simulink model "Lane_Keep_Assist"  (R2025a)
settings: Solver=VariableStepAuto  StartTime=0.0  StopTime=10.0  RelTol=1e-3
libraries: slpidlib x1
settings Model: Creator=Rudransh  LastModifiedBy=Rudransh

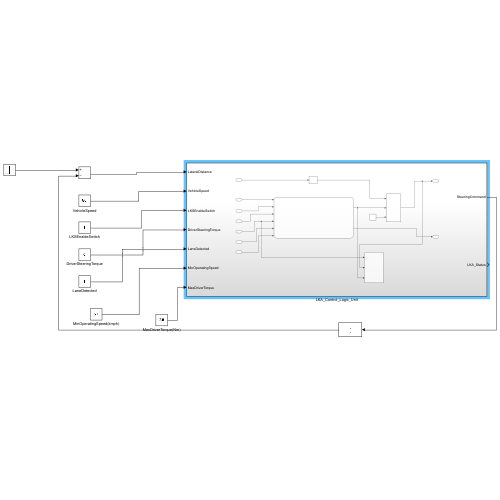
[thumbnail: Simulink's stored preview of the top-level diagram]
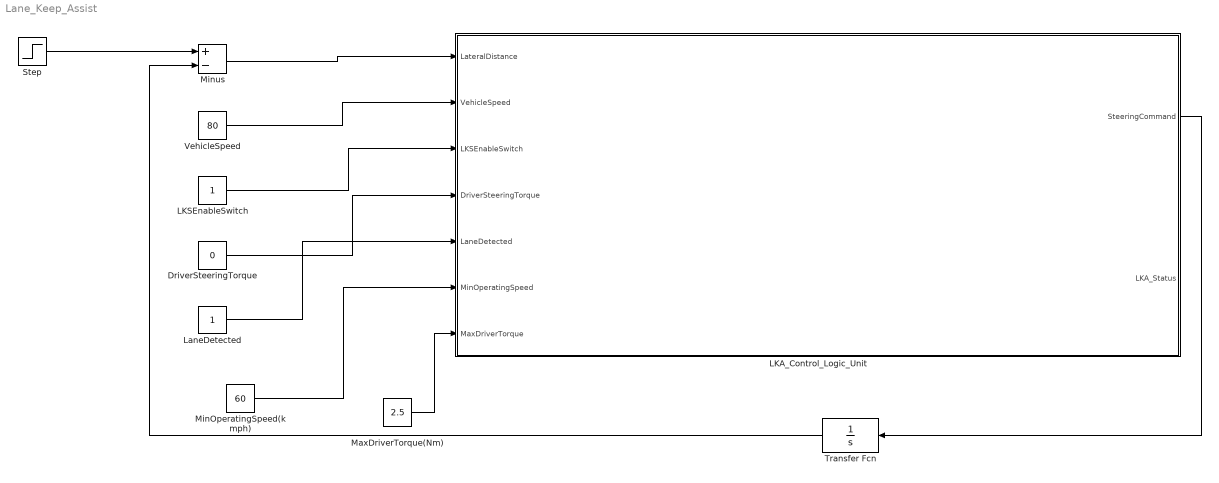
== system Lane_Keep_Assist ==
  DriverSteeringTorque : Constant  Value=0
  LKA_Control_Logic_Unit : Subsystem
  LKSEnableSwitch : Constant
  LaneDetected : Constant
  MaxDriverTorque(Nm) : Constant  Value=2.5
  MinOperatingSpeed(kmph) : Constant  Value=60
  Minus : Sum  Inputs=+-
  Step : Step  After=0.5  SampleTime=0
  Transfer Fcn : TransferFcn  Denominator=[1 0]
  VehicleSpeed : Constant  Value=80
  wires:
  LaneDetected/1 -> LKA_Control_Logic_Unit/5(LaneDetected)
  DriverSteeringTorque/1 -> LKA_Control_Logic_Unit/4(DriverSteeringTorque)
  LKSEnableSwitch/1 -> LKA_Control_Logic_Unit/3(LKSEnableSwitch)
  VehicleSpeed/1 -> LKA_Control_Logic_Unit/2(VehicleSpeed)
  Minus/1 -> LKA_Control_Logic_Unit/1(LateralDistance)
  LKA_Control_Logic_Unit/1(SteeringCommand) -> Transfer Fcn/1
  Transfer Fcn/1 -> Minus/2
  MaxDriverTorque(Nm)/1 -> LKA_Control_Logic_Unit/7(MaxDriverTorque)
  MinOperatingSpeed(kmph)/1 -> LKA_Control_Logic_Unit/6(MinOperatingSpeed)
  Step/1 -> Minus/1

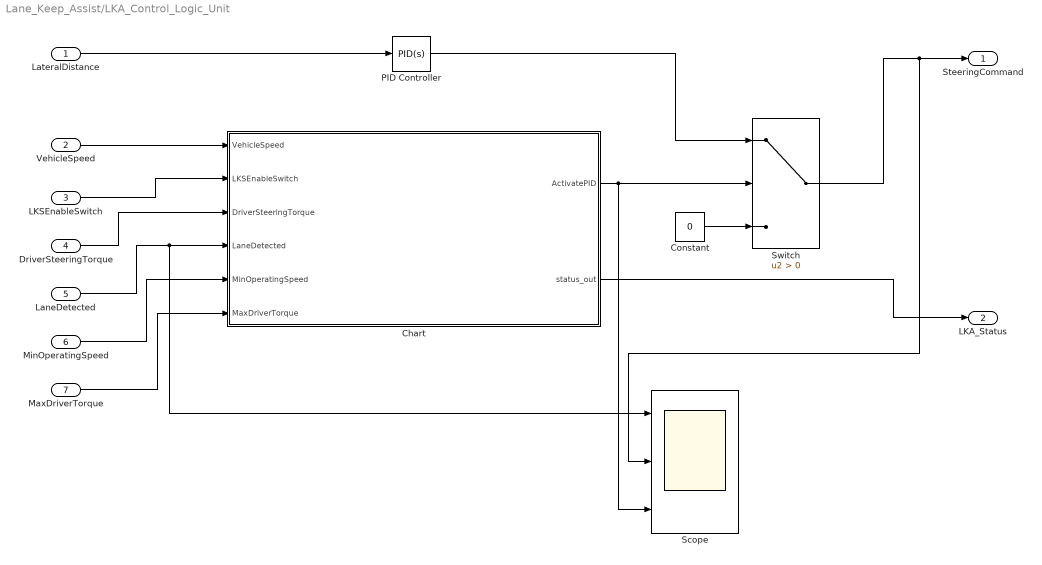
== system Lane_Keep_Assist/LKA_Control_Logic_Unit ==
  LateralDistance : Inport
  VehicleSpeed : Inport  Port=2
  LKSEnableSwitch : Inport  Port=3
  DriverSteeringTorque : Inport  Port=4
  LaneDetected : Inport  Port=5
  MinOperatingSpeed : Inport  Port=6
  MaxDriverTorque : Inport  Port=7  PortDimensions=1
  Chart : Stateflow chart  TreatAsAtomicUnit=on
  Constant : Constant  Value=0
  PID Controller : slpidlib/PID Controller  Controller=PID  Form=Parallel  TimeDomain=Continuous-time  UseExternalTs=off  SampleTime=-1  IntegratorMethod=Forward Euler  FilterMethod=Forward Euler  ControllerParametersSource=internal  P=60  I=5  UseKiTs=off  D=120  UseExternalDerivativeSource=off  N=100  UseFilter=on  TunerSelectOption=Transfer Function Based (PID Tuner App)  InitialConditionSource=internal  InitialConditionForIntegrator=0  InitialConditionForFilter=0  DifferentiatorICPrevScaledInput=0  ExternalReset=none  TrackingMode=off  Kt=1  LimitOutput=on  SatLimitsSource=internal  UpperSaturationLimit=5  LowerSaturationLimit=-5  LinearizeAsGain=on  AntiWindupMode=none  Kb=1  LimitIntegrator=off  UpperIntegratorSaturationLimit=inf  LowerIntegratorSaturationLimit=-inf  POutMin=[]  POutMax=[]  IOutMin=[]  IOutMax=[]  DOutMin=[]  DOutMax=[]  NOutMin=[]  NOutMax=[]  SumOutMin=[]  SumOutMax=[]  SaturationOutMin=[]  SaturationOutMax=[]  PParamMin=[]  PParamMax=[]  IParamMin=[]  IParamMax=[]  DParamMin=[]  DParamMax=[]  NParamMin=[]  NParamMax=[]  KbParamMin=[]  KbParamMax=[]  KtParamMin=[]  KtParamMax=[]  KbOutMin=[]  KbOutMax=[]  KtOutMin=[]  KtOutMax=[]  IntegratorOutMin=[]  IntegratorOutMax=[]  FilterOutMin=[]  FilterOutMax=[]  SumI1OutMin=[]  SumI1OutMax=[]  SumI2OutMin=[]  SumI2OutMax=[]  SumI3OutMin=[]  SumI3OutMax=[]  SumI4OutMin=[]  SumI4OutMax=[]  SumDOutMin=[]  SumDOutMax=[]  DifferentiatorOutMin=[]  DifferentiatorOutMax=[]  FilterDiffOutCoefMin=[]  FilterDiffOutCoefMax=[]  ReciprocalOutMin=[]  ReciprocalOutMax=[]  SumDenOutMin=[]  SumDenOutMax=[]  SumNumOutMin=[]  SumNumOutMax=[]  DivideOutMin=[]  DivideOutMax=[]  UdiffTsProdOutMin=[]  UdiffTsProdOutMax=[]  NTsProdOutMin=[]  NTsProdOutMax=[]  UintegralTsProdOutMin=[]  UintegralTsProdOutMax=[]  UngainTsProdOutMin=[]  UngainTsProdOutMax=[]  ClampingZeroOutDataTypeStr=Inherit: Inherit via back propagation  ClampingZeroOutMin=[]  ClampingZeroOutMax=[]  FilterDenConstantOutDataTypeStr=Inherit: Inherit via back propagation  FilterDenConstantOutMin=[]  FilterDenConstantOutMax=[]  PCopyOutDataTypeStr=Inherit: Inherit via back propagation  PCopyOutMin=[]  PCopyOutMax=[]  NCopyOutDataTypeStr=Inherit: Inherit via back propagation  NCopyOutMin=[]  NCopyOutMax=[]  IntegratorContinuousStateAttributes=''  IntegratorStateMustResolveToSignalObject=off  IntegratorRTWStateStorageClass=Auto  FilterContinuousStateAttributes=''  FilterStateMustResolveToSignalObject=off  FilterRTWStateStorageClass=Auto  ParallelPVariant=InternalParameters  IdealPVariant=Disabled  IVariant=InternalParameters  DVariant=InternalParameters  IntegratorVariant=Continuous  SatVariant=Enabled  AWVariant=Passthrough  PCopyVariant=Disabled  TRVariant=Disabled  FdbkBlocksVariant=Forward  IdealPFdbkVariant=Disabled  SatFdbkVariant=Disabled  DerivativeFilterVariant=ContFilter  NVariant=InternalParameters  NCopyVariant=Disabled  FilterICVariant=InternalICsFilter  IntegratorICVariant=InternalICs  ExternalResetVariant=Disabled  TRSumVariant=Passthrough  SumFdbkVariant=Disabled  SumVariant=Sum_PID  TsampFilterVariant=InternalTs  TsampNgainVariant=Passthrough  TsampIntegralVariant=Disabled_SignalSpec  ExternalSaturationOutDataTypeStr=Inherit: Same as second input  DerivativeSourceVariant=ErrorSignal  PreIntVariant=InternalPreInt
  Scope : Scope  NumInputPorts=3
      settings: ActiveDisplayString=3  Title=LKAStatus  ActiveDisplayYMinimum=0  ActiveDisplayYMaximum=1
  Switch : Switch  Criteria=u2 > Threshold  SaturateOnIntegerOverflow=off  InputSameDT=off
  SteeringCommand : Outport
  LKA_Status : Outport  Port=2
  wires:
  VehicleSpeed/1 -> Chart/1(VehicleSpeed)
  LKSEnableSwitch/1 -> Chart/2(LKSEnableSwitch)
  DriverSteeringTorque/1 -> Chart/3(DriverSteeringTorque)
  LaneDetected/1 -> Scope/1, Chart/4(LaneDetected)
  LateralDistance/1 -> PID Controller/1
  Chart/1(ActivatePID) -> Scope/3, Switch/2
  PID Controller/1 -> Switch/1
  Constant/1 -> Switch/3
  Switch/1 -> Scope/2, SteeringCommand/1
  Chart/2(status_out) -> LKA_Status/1
  MinOperatingSpeed/1 -> Chart/5(MinOperatingSpeed)
  MaxDriverTorque/1 -> Chart/6(MaxDriverTorque)

== stateflow chart Lane_Keep_Assist/LKA_Control_Logic_Unit/Chart ==
  state OFF
    status_out = OFF;
    ActivatePID = 0;
  state PASSIVE
    status_out = PASSIVE;
    ActivatePID = 0;
  state ACTIVE
    status_out = ACTIVE;
    ActivatePID = 1;
  state OVERRIDE
    status_out = OVERRIDE;
    ActivatePID = 0;
  OVERRIDE -> OFF [order 2] : [LKSEnableSwitch == 0]
  (default) -> OFF
  OFF -> PASSIVE : [LKSEnableSwitch == 1]
  ACTIVE -> OFF [order 3] : [LKSEnableSwitch == 0]
  PASSIVE -> OFF [order 1] : [LKSEnableSwitch == 0]
  PASSIVE -> ACTIVE [order 2] : [VehicleSpeed >= MinOperatingSpeed && LaneDetected == 1]
  ACTIVE -> PASSIVE [order 1] : [VehicleSpeed < MinOperatingSpeed || LaneDetected == 0]
  ACTIVE -> OVERRIDE [order 2] : [abs(DriverSteeringTorque) > MaxDriverTorque]
  OVERRIDE -> ACTIVE [order 1] : [abs(DriverSteeringTorque) <= MaxDriverTorque]
  data: VehicleSpeed input; LKSEnableSwitch input; DriverSteeringTorque input; LaneDetected input; ActivatePID output; status_out output; MinOperatingSpeed input; MaxDriverTorque input
  events: OFF local FUNCTION_CALL_EVENT; PASSIVE local FUNCTION_CALL_EVENT; ACTIVE local FUNCTION_CALL_EVENT; OVERRIDE local FUNCTION_CALL_EVENT
